simulink model "kinematics_simulaink "  (R2019a)
settings: Solver=VariableStepAuto  StartTime=0.0  StopTime=10.0  RelTol=1e-3
libraries: simulink_extras x4
settings Model: Creator=Ashraf  LastModifiedBy=Ashraf

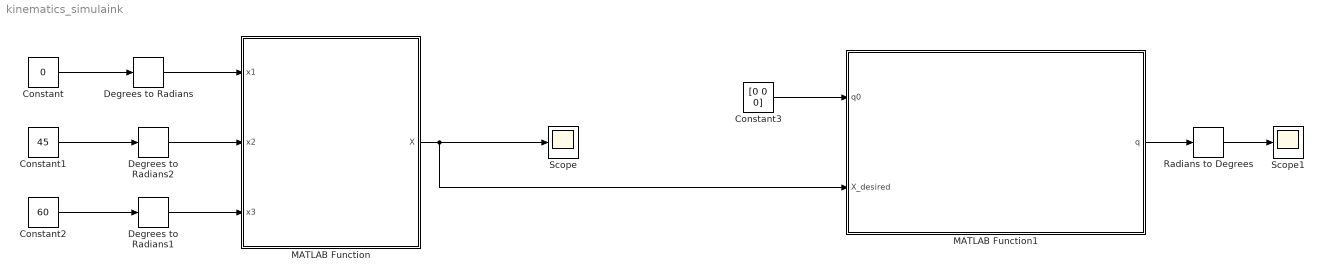
== system kinematics_simulaink  ==
  Constant : Constant  Value=0
  Constant1 : Constant  Value=45
  Constant2 : Constant  Value=60
  Constant3 : Constant  Value=[0 0 0]
  Degrees to Radians : simulink_extras/Transformations/Degrees to Radians
  Degrees to Radians1 : simulink_extras/Transformations/Degrees to Radians
  Degrees to Radians2 : simulink_extras/Transformations/Degrees to Radians
  MATLAB Function : MATLAB Function  TreatAsAtomicUnit=on
  MATLAB Function1 : MATLAB Function  TreatAsAtomicUnit=on
  Radians to Degrees : simulink_extras/Transformations/Radians to Degrees
  Scope : Scope
  Scope1 : Scope
  wires:
  MATLAB Function/1(X) -> MATLAB Function1/2(X_desired), Scope/1
  Constant3/1 -> MATLAB Function1/1(q0)
  Degrees to Radians/1 -> MATLAB Function/1(x1)
  Constant/1 -> Degrees to Radians/1
  Constant1/1 -> Degrees to Radians2/1
  Degrees to Radians2/1 -> MATLAB Function/2(x2)
  Degrees to Radians1/1 -> MATLAB Function/3(x3)
  Constant2/1 -> Degrees to Radians1/1
  MATLAB Function1/1(q) -> Radians to Degrees/1
  Radians to Degrees/1 -> Scope1/1

== matlab function kinematics_simulaink /MATLAB Function1 ==
  data: q0 input; q output; X_desired input
function q = inverse_kinematics_func(q0, X_desired)
    tolerance = 1e-6;
    max_iterations = 100;
    q = q0; % Initial guess for joint angles

    for i = 1:max_iterations
        % Compute forward kinematics with current q
        DH_table = [
            q(1), 100, -15, pi/2;
            q(2), 0, 120, 0;
            q(3), 0, 120, 0
        ];
        X_current = forward_kinematics_func(DH_table);

        % Calculate error
        error = X_desired - X_current;
        
        % Break if error is within tolerance
        if norm(error) < tolerance
            break;
        end

        % Compute inverse Jacobian
        J_inv = inverse_jacobian_matrix(q);

        % Update joint angles
        q = q + J_inv * error;
    end
end   

% Forward kinematics function
function X = forward_kinematics_func(DH_table)
    T_total = eye(4);
    for i = 1:size(DH_table, 1)
        theta = DH_table(i, 1);  
        d = DH_table(i, 2);      
        a = DH_table(i, 3);      
        alpha = DH_table(i, 4);  
        T = transformation_func(theta, d, a, alpha);
        T_total = T_total * T;
    end
    X = T_total(1:3, 4); % Extract end-effector position
end

% Transformation matrix function
function T = transformation_func(theta, d, a, alpha)
    T = [cos(theta), -sin(theta)*cos(alpha), sin(theta)*sin(alpha), a*cos(theta);
         sin(theta), cos(theta)*cos(alpha),  -cos(theta)*sin(alpha), a*sin(theta);
         0,          sin(alpha),            cos(alpha),            d;
         0,          0,                     0,                     1];
end

% Inverse Jacobian function without symbolic operations
function J_inv = inverse_jacobian_matrix(q)
    % Extract joint angles
    q1 = q(1);
    q2 = q(2);
    q3 = q(3);

    % Define DH parameters numerically
    l0 = 100; 
    l1 = 120;
    l2 = 120;

    % Numerically compute the Jacobian matrix
    J = zeros(3, 3);  % Initialize Jacobian as a numeric array
    epsilon = 1e-6;   % Small value for numerical differentiation

    % Compute partial derivatives of the end-effector position
    for i = 1:3
        q_plus = q;
        q_plus(i) = q_plus(i) + epsilon;  % Perturb each joint variable
        
        DH_table_plus = [
            q_plus(1), l0, -15, pi/2;
            q_plus(2), 0, l1, 0;
            q_plus(3), 0, l2, 0
        ];
        
        % Forward kinematics with perturbed angle
        X_plus = forward_kinematics_func(DH_table_plus);
        
        % Forward kinematics with original angle
        DH_table = [
            q1, l0, -15, pi/2;
            q2, 0, l1, 0;
            q3, 0, l2, 0
        ];
        X = forward_kinematics_func(DH_table);

        % Numerical derivative
        J(:, i) = (X_plus - X) / epsilon;
    end

    % Compute inverse or pseudo-inverse based on Jacobian rank
    if rank(J) == size(J, 1)
        J_inv = inv(J); % Exact inverse
    else
        J_inv = pinv(J); % Pseudo-inverse
    end
end

== matlab function kinematics_simulaink /MATLAB Function ==
  data: x1 input; X output; x2 input; x3 input
function X = forward_kinematics_func(x1,x2,x3)
    l0 = 100; 
    l1 = 120;
    l2 = 120;
    l3 = 42.16;


    % DH Table for forward kinematics
    DH_table = [
        x1, l0, -15, pi/2;
        x2, 0, l1, 0;
        x3, 0, l2, 0
    ];
    T_total = eye(4);
    for i = 1:size(DH_table, 1)
        theta = DH_table(i, 1);  
        d = DH_table(i, 2);      
        a = DH_table(i, 3);      
        alpha = DH_table(i, 4);  
        T = transformation_func(theta, d, a, alpha);
        T_total = T_total * T;
    end
    X = T_total(1:3, 4); % Extract end-effector position
end

function T = transformation_func(theta, d, a, alpha)
    T = [cos(theta), -sin(theta)*cos(alpha), sin(theta)*sin(alpha), a*cos(theta);
         sin(theta), cos(theta)*cos(alpha),  -cos(theta)*sin(alpha), a*sin(theta);
         0,          sin(alpha),            cos(alpha),            d;
         0,          0,                     0,                     1];
end
